simulink model "velo_pi_mbd_sl"  (Simulink 7.9)
settings: Solver=ode4  StartTime=0.0  StopTime=20  RelTol=1e-3
values from neighbouring files (symbols this model uses):
  K = 1.57    [model_data.mat]    (also in velo_id_verify.m)
  Ki = p1*p2*T/K    [velo_pi_mbd.m]
  Kp = -((p1+p2)*T + 1)/K    [velo_pi_mbd.m]
  T = 0.76    [model_data.mat]    (also in velo_id_verify.m)
  ts = 1/50    (= 0.02)    [velo_id_gain.m]    (also in velo_id_tc.m; velo_pi_mbd.m)
  u_offset = 1.03    [model_data.mat]    (also in velo_id_gain.m = -P(2)/P(1); velo_id_tc.m = (K_id*r_const -c1)/K_id; velo_id_verify.m)
libraries: arduino_io_lib x4
settings Model: Creator=hirata  LastModifiedBy=hirata

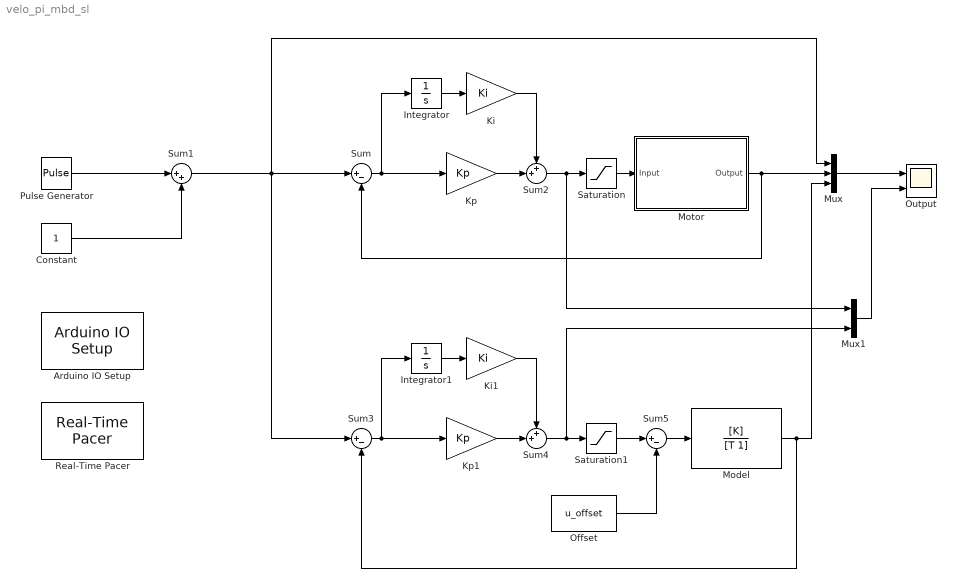
== system velo_pi_mbd_sl ==
  Arduino IO Setup : arduino_io_lib/Arduino IO Setup  Priority=3  arduinoVar=Arduino1  comPort=COM3
  Constant : Constant
  Integrator : Integrator
  Integrator1 : Integrator
  Ki : Gain  Gain=Ki
  Ki1 : Gain  Gain=Ki
  Kp : Gain  Gain=Kp
  Kp1 : Gain  Gain=Kp
  Model : TransferFcn  Numerator=[K]  Denominator=[T 1]
  Motor : Subsystem
  Mux : Mux  Inputs=3
  Mux1 : Mux  Inputs=2
  Offset : Constant  Value=u_offset
  Output : Scope  NumInputPorts=2
      settings: TimeRange=10  YMin=0.5~0  YMax=2~5
  Pulse Generator : DiscretePulseGenerator  Amplitude=0.5  Period=4/ts  PulseWidth=2/ts  SampleTime=ts
  Real-Time Pacer : arduino_io_lib/Real-Time Pacer  simTimePerRealTime=1
  Saturation : Saturate  UpperLimit=5  LowerLimit=0
  Saturation1 : Saturate  UpperLimit=5  LowerLimit=0
  Sum : Sum  Inputs=|+-
  Sum1 : Sum  Inputs=|++
  Sum2 : Sum  Inputs=++|
  Sum3 : Sum  Inputs=|+-
  Sum4 : Sum  Inputs=++|
  Sum5 : Sum  Inputs=|+-
  wires:
  Motor/1(Output) -> Mux/2, Sum/2
  Mux/1 -> Output/1
  Sum2/1 -> Mux1/1, Saturation/1
  Sum/1 -> Kp/1, Integrator/1
  Constant/1 -> Sum1/2
  Pulse Generator/1 -> Sum1/1
  Sum1/1 -> Sum/1, Sum3/1, Mux/1
  Integrator/1 -> Ki/1
  Ki/1 -> Sum2/1
  Kp/1 -> Sum2/2
  Model/1 -> Sum3/2, Mux/3
  Sum4/1 -> Mux1/2, Saturation1/1
  Sum3/1 -> Kp1/1, Integrator1/1
  Integrator1/1 -> Ki1/1
  Ki1/1 -> Sum4/1
  Kp1/1 -> Sum4/2
  Mux1/1 -> Output/2
  Saturation/1 -> Motor/1(Input)
  Saturation1/1 -> Sum5/1
  Sum5/1 -> Model/1
  Offset/1 -> Sum5/2

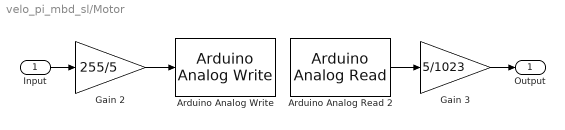
== system velo_pi_mbd_sl/Motor ==
  Input : Inport
  Arduino Analog Read 2 : arduino_io_lib/Arduino Analog Read  arduinoVar=Arduino1  arduinoPin=0  T=ts
  Arduino Analog Write : arduino_io_lib/Arduino Analog Write  arduinoVar=Arduino1  arduinoPin=3  T=ts
  Gain 2 : Gain  Gain=255/5
  Gain 3 : Gain  Gain=5/1023
  Output : Outport
  wires:
  Arduino Analog Read 2/1 -> Gain 3/1
  Gain 2/1 -> Arduino Analog Write/1
  Input/1 -> Gain 2/1
  Gain 3/1 -> Output/1
